simulink model "RoadTestingDynamic"  (Simulink 7.9)
settings: Solver=ode45  StartTime=0.0  StopTime=10.0  RelTol=1e-3
PostLoadFcn:
  | Threshold = 8;
  | MaxCluster = 25;
  | Num_Beams = 726;
  | Road_Width = 8.5;
  | Cone_Width = .015;
  | Scaling = 1;
  | javaaddpath({'/'});
  | import ClusterMethodWithRoadDynamic.*;
  | import Geometry.*;
  | DataCluster = ClusterMethodWithRoadDynamic(Threshold,MaxCluster,Scaling,Road_Width,Cone_Width);
  | eml.extrinsic('evalin');
undefined symbols (not defined in the file or in its folder): Run_11
settings Model: Creator=Thomas  LastModifiedBy=TCA
settings DataIOCC: SignalLoggingSaveFormat=Dataset

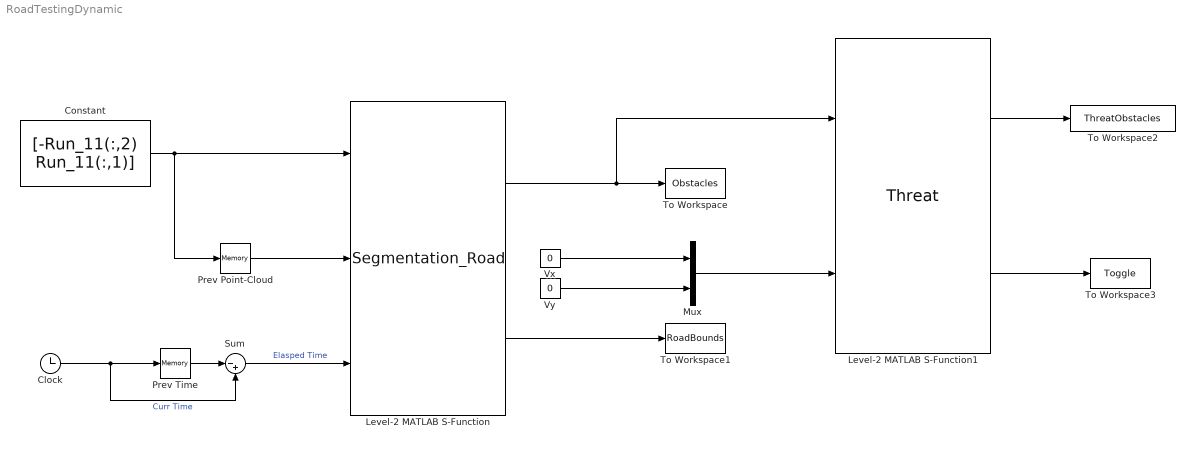
== system RoadTestingDynamic ==
  Clock : Clock
  Constant : Constant  Value=[-Run_11(:,2) Run_11(:,1)]
  Level-2 MATLAB S-Function : M-S-Function  FunctionName=Segmentation_Road
  Level-2 MATLAB S-Function1 : M-S-Function  FunctionName=Threat  Parameters=0.25,10,1
  Mux : Mux  Inputs=2
  Prev Point-Cloud : Memory
  Prev Time : Memory
  Sum : Sum  Inputs=|-+
  To Workspace : ToWorkspace  VariableName=Obstacles  SampleTime=-1  SaveFormat=Structure With Time
  To Workspace1 : ToWorkspace  VariableName=RoadBounds  SampleTime=-1
  To Workspace2 : ToWorkspace  VariableName=ThreatObstacles  SampleTime=-1  SaveFormat=Structure With Time
  To Workspace3 : ToWorkspace  VariableName=Toggle  SampleTime=-1
  Vx : Constant  Value=0
  Vy : Constant  Value=0
  wires:
  Prev Time/1 -> Sum/1
  Sum/1 -> Level-2 MATLAB S-Function/3  "Elasped Time"
  Clock/1 -> Prev Time/1, Sum/2  "Curr Time"
  Prev Point-Cloud/1 -> Level-2 MATLAB S-Function/2
  Constant/1 -> Prev Point-Cloud/1, Level-2 MATLAB S-Function/1
  Level-2 MATLAB S-Function/1 -> Level-2 MATLAB S-Function1/1, To Workspace/1
  Level-2 MATLAB S-Function/2 -> To Workspace1/1
  Vx/1 -> Mux/1
  Mux/1 -> Level-2 MATLAB S-Function1/2
  Level-2 MATLAB S-Function1/1 -> To Workspace2/1
  Level-2 MATLAB S-Function1/2 -> To Workspace3/1
  Vy/1 -> Mux/2
